simulink model "SMA_displacementIn"  (R2016a)
settings: Solver=ode15s  StartTime=0.0  StopTime=100  RelTol=1e-6  AbsTol=1e-6
InitFcn:
  | Parameter;
values from neighbouring files (symbols this model uses):
  params = block.DialogPrm(1).Data    [sDE_dispIn.m]    (also in sSMA_displacementIn.m)
libraries: simulink x1
settings Model: Creator=Johannes  LastModifiedBy=Gianluca
settings DataIOCC: LimitDataPoints=on  SaveFormat=Array  SignalLoggingSaveFormat=ModelDataLogs
settings DebuggingCC: UnderspecifiedInitializationDetection=Classic  MergeDetectMultiDrivingBlocksExec=none  SolverPrmCheckMsg=warning  MultiTaskDSMMsg=warning  MultiTaskCondExecSysMsg=none
settings HardwareCC: ProdBitPerPointer=32  ProdLargestAtomicFloat=None  ProdIntDivRoundTo=Undefined  ProdEndianess=Unspecified  ProdWordSize=32  ProdHWDeviceType=32-bit Generic
settings ModelReferenceCC: PropagateSignalLabelsOutOfModel=off
settings ConfigComp: CovModelRefEnable=Off

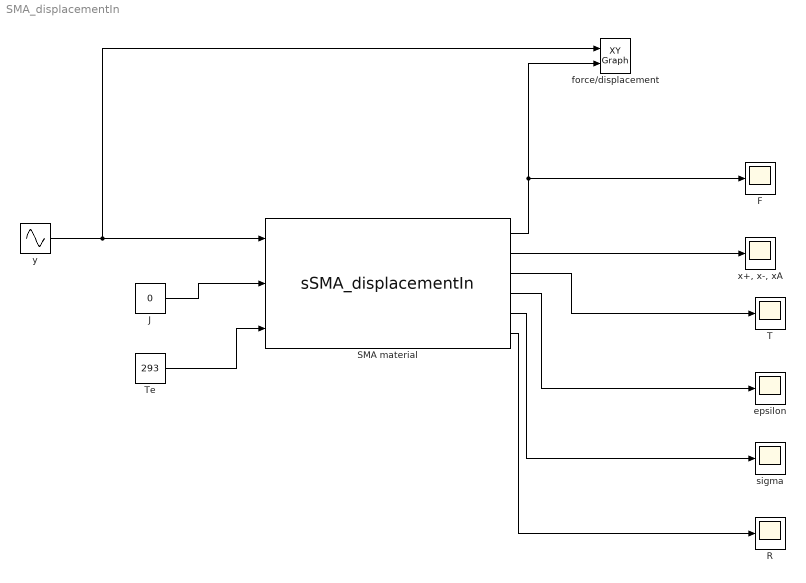
== system SMA_displacementIn ==
  F : Scope
  J : Constant  Value=0
  R : Scope
  SMA material : M-S-Function  FunctionName=sSMA_displacementIn  Parameters=params, initConds
      mask Display:
      | color('black');
      | patch(3*[-1 1 1 -1],1.1*[-1 -1 1 1],[1 1 1]);
      | patch([-1.6 -0.8],[-0.9 0.3],[0 0 0]);
      | patch([-0.8 1.2],[0.3 0.3],[0 0 0]);
      | patch([1.6 0.8],[0.9 -0.3],[0 0 0]);
      | patch([0.8 -1.2],[-0.3 -0.3],[0 0 0]);
      | disp('SMA');
      | 
      | color('blue');
      | port_label('input', 1, 'y [m]','texmode','on');
      | port_label('input', 2, 'J [W]','texmode','on');
      | port_label('input', 3, 'T_E [K]','texmode','on');
      | 
      | color('red');
      | port_label('output', 1, 'F [N]','texmode','on');
      | port_label('output', 2, 'x_+, x_-, x_A [-]','texmode','on');
      | port_label('output', 3, 'T [K]','texmode','on');
      | port_label('output', 4, '\epsilon [-]','texmode','on');
      | port_label('output', 5, '\sigma [Pa]','texmode','on');
      | port_label('output', 6, 'R [\Omega]','texmode','on');
  T : Scope
  Te : Constant  Value=293
  epsilon : Scope
  force/displacement : simulink/Sinks/XY Graph  xmin=0.1  xmax=0.107  ymin=0  ymax=5  st=-1
  sigma : Scope
  "x+, x-, xA" : Scope
  y : Sin  Amplitude=0.035*params.L0  Bias=params.L0*1.035  Frequency=2*pi/100  Phase=-pi/2  SampleTime=0
  wires:
  J/1 -> SMA material/2
  Te/1 -> SMA material/3
  SMA material/1 -> F/1, force/displacement/2
  SMA material/2 -> "x+, x-, xA"/1
  SMA material/3 -> T/1
  SMA material/4 -> epsilon/1
  SMA material/5 -> sigma/1
  SMA material/6 -> R/1
  y/1 -> force/displacement/1, SMA material/1
